simulink model "Simulacion"  (R2020a)
settings: Solver=VariableStepAuto  StartTime=0.0  StopTime=2  RelTol=1e-3
settings Model: Creator=Miguel Gutierrez  LastModifiedBy=Miguel Gutierrez

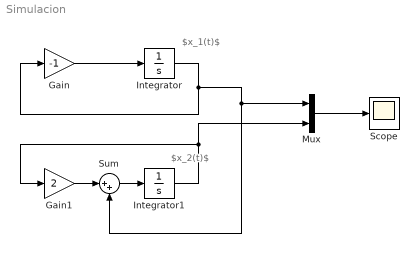
== system Simulacion ==
  note: $x_1(t)$
  note: $x_2(t)$
  Gain : Gain  Gain=-1
  Gain1 : Gain  Gain=2
  Integrator : Integrator  InitialCondition=1
  Integrator1 : Integrator  InitialCondition=1
  Mux : Mux  Inputs=2
  Scope : Scope
  Sum : Sum  Inputs=|++
  wires:
  Gain/1 -> Integrator/1
  Integrator1/1 -> Mux/2, Gain1/1
  Gain1/1 -> Sum/1
  Sum/1 -> Integrator1/1
  Integrator/1 -> Mux/1, Sum/2, Gain/1
  Mux/1 -> Scope/1
